simulink model "SF104A_MotCurrRegCfg"  (R2013b)
settings: Solver=FixedStepDiscrete  SolverMode=SingleTasking  StartTime=0.0  StopTime=1  FixedStep=0.002  RelTol=1e-3
values from neighbouring files (symbols this model uses):
  ARCHGLBPRM_2MILLISEC_SEC_F32 = DataDict.Constant    [SF104A_MotCurrRegCfg_DataDict.m]
  ARCHGLBPRM_2PI_ULS_F32 = DataDict.Constant    [SF104A_MotCurrRegCfg_DataDict.m]
  ARCHGLBPRM_HALFSQRT3_ULS_F32 = DataDict.Constant    [SF104A_MotCurrRegCfg_DataDict.m]
  MotCurrRegCfgCtrlrDynGainVehSpdCutOff = DataDict.Calibration    [SF104A_MotCurrRegCfg_DataDict.m]
  MotCurrRegCfgCurrLoopSecOrderTrfFctEna = DataDict.Calibration    [SF104A_MotCurrRegCfg_DataDict.m]
  MotCurrRegCfgIntglGainSampleTi = DataDict.Calibration    [SF104A_MotCurrRegCfg_DataDict.m]
  MotCurrRegCfgMotAgCompuDly = DataDict.Calibration    [SF104A_MotCurrRegCfg_DataDict.m]
  MotCurrRegCfgMotClsdLoopBwDaxY = DataDict.Calibration    [SF104A_MotCurrRegCfg_DataDict.m]
  MotCurrRegCfgMotClsdLoopBwQaxY = DataDict.Calibration    [SF104A_MotCurrRegCfg_DataDict.m]
  MotCurrRegCfgMotDampgRatDax = DataDict.Calibration    [SF104A_MotCurrRegCfg_DataDict.m]
  MotCurrRegCfgMotDampgRatQax = DataDict.Calibration    [SF104A_MotCurrRegCfg_DataDict.m]
  MotCurrRegCfgMotNatFrqDaxY = DataDict.Calibration    [SF104A_MotCurrRegCfg_DataDict.m]
  MotCurrRegCfgMotNatFrqQaxY = DataDict.Calibration    [SF104A_MotCurrRegCfg_DataDict.m]
  MotCurrRegCfgMotRVirtDax = DataDict.Calibration    [SF104A_MotCurrRegCfg_DataDict.m]
  MotCurrRegCfgMotRVirtQax = DataDict.Calibration    [SF104A_MotCurrRegCfg_DataDict.m]
  MOTDAMPGRATCON_ULS_F32 = DataDict.Constant    [SF104A_MotCurrRegCfg_DataDict.m]
  MotRefMdlFbCtrlDi = DataDict.ImprtdCal    [SF104A_MotCurrRegCfg_DataDict.m]
  POLETOPHA_ULS_F32 = DataDict.Constant    [SF104A_MotCurrRegCfg_DataDict.m]
  SysGlbPrmMotPoleCnt = DataDict.ImprtdCal    [SF104A_MotCurrRegCfg_DataDict.m]
  ZEROMOTCTRLGAIN_OHM_F32 = DataDict.Constant    [SF104A_MotCurrRegCfg_DataDict.m]
undefined symbols (not defined in the file or in its folder): MotCurrEolCalSt2
libraries: NxtrLim x11, FixdToFloat x4, LnrIntrpn x4, simulink x3, Fil x2, FloatToFixd x1
(part 3 of 3)

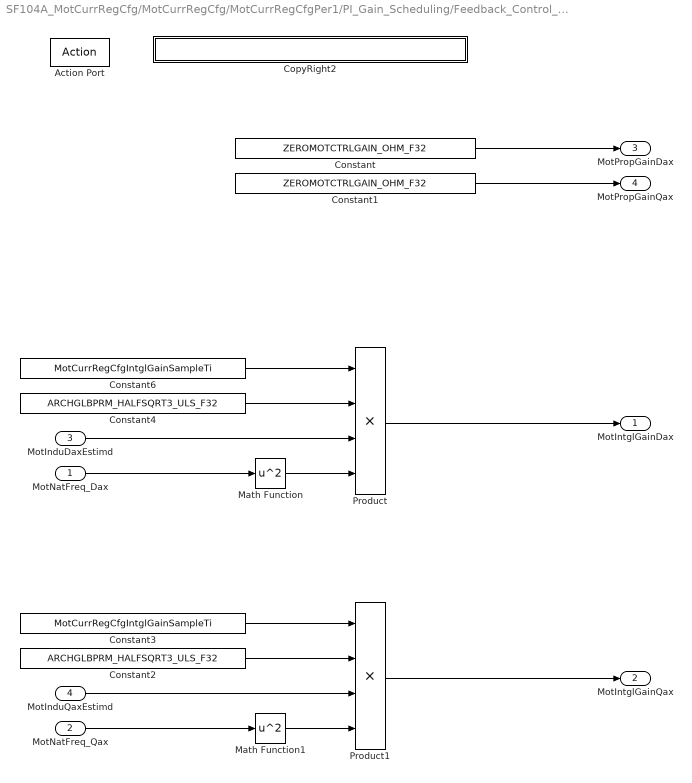
== system SF104A_MotCurrRegCfg/MotCurrRegCfg/MotCurrRegCfgPer1/PI_Gain_Scheduling/Feedback_Control_ Enabled/Calculate_Gains/2nd Order Enabled ==
  MotNatFreq_Dax : Inport  RequirementInfo="{'linktype_rmi_doors' '0000bb43 (/E-STEER Core/SubSystem Specifications/Application Functions/SF99/SF104A Current Regulator Configuration)' '#SF104A_102' 'true' 'REQ:  SF104A_102' '' } %GIDa_3ffef093_6233_4daa_8141_5ade26bfe0b7"
  MotNatFreq_Qax : Inport  RequirementInfo="{'linktype_rmi_doors' '0000bb43 (/E-STEER Core/SubSystem Specifications/Application Functions/SF99/SF104A Current Regulator Configuration)' '#SF104A_102' 'true' 'REQ:  SF104A_102' '' } %GIDa_0729f0b0_64c3_4f7f_a23b_323a26491a45"  Port=2
  MotInduDaxEstimd : Inport  RequirementInfo="{'linktype_rmi_doors' '0000bb43 (/E-STEER Core/SubSystem Specifications/Application Functions/SF99/SF104A Current Regulator Configuration)' '#SF104A_102' 'true' 'REQ:  SF104A_102' '' } %GIDa_89f11cc6_5f7a_4c49_9846_35a9922d5407"  Port=3
  MotInduQaxEstimd : Inport  RequirementInfo="{'linktype_rmi_doors' '0000bb43 (/E-STEER Core/SubSystem Specifications/Application Functions/SF99/SF104A Current Regulator Configuration)' '#SF104A_102' 'true' 'REQ:  SF104A_102' '' } %GIDa_2fe3e424_844e_4ee7_a315_46d12420253b"  Port=4
  Action Port : ActionPort  ActionType=then
  Constant : Constant  RequirementInfo="{'linktype_rmi_doors' '0000bb43 (/E-STEER Core/SubSystem Specifications/Application Functions/SF99/SF104A Current Regulator Configuration)' '#SF104A_102' 'true' 'REQ:  SF104A_102' '' } %GIDa_5901fc89_50da_4871_894f_d7a4bc965ae3"  Value=ZEROMOTCTRLGAIN_OHM_F32  OutDataTypeStr=single
  Constant1 : Constant  RequirementInfo="{'linktype_rmi_doors' '0000bb43 (/E-STEER Core/SubSystem Specifications/Application Functions/SF99/SF104A Current Regulator Configuration)' '#SF104A_102' 'true' 'REQ:  SF104A_102' '' } %GIDa_5a773f90_f553_49c4_87dd_9299d647398d"  Value=ZEROMOTCTRLGAIN_OHM_F32  OutDataTypeStr=single
  Constant2 : Constant  RequirementInfo="{'linktype_rmi_doors' '0000bb43 (/E-STEER Core/SubSystem Specifications/Application Functions/SF99/SF104A Current Regulator Configuration)' '#SF104A_102' 'true' 'REQ:  SF104A_102' '' } %GIDa_a4f8ec7f_a439_41cb_b2c0_2d5eeb2fedbe"  Value=ARCHGLBPRM_HALFSQRT3_ULS_F32
  Constant3 : Constant  RequirementInfo="{'linktype_rmi_doors' '0000bb43 (/E-STEER Core/SubSystem Specifications/Application Functions/SF99/SF104A Current Regulator Configuration)' '#SF104A_118' 'true' 'REQ:  SF104A_118' '' ; 'linktype_rmi_doors' '0000bb43 (/E-STEER Core/SubSystem Specifications/Application Functions/SF99/SF104A Current Regulator Configuration)' '#SF104A_102' 'true' 'REQ:  SF104A_102' '' } %GIDa_714edeba_1674_4f10_b7a8_b0e92a37ae0d"  Value=MotCurrRegCfgIntglGainSampleTi
  Constant4 : Constant  RequirementInfo="{'linktype_rmi_doors' '0000bb43 (/E-STEER Core/SubSystem Specifications/Application Functions/SF99/SF104A Current Regulator Configuration)' '#SF104A_102' 'true' 'REQ:  SF104A_102' '' } %GIDa_0619ee1d_6818_4fb5_9ced_1ceae65db526"  Value=ARCHGLBPRM_HALFSQRT3_ULS_F32
  Constant6 : Constant  RequirementInfo="{'linktype_rmi_doors' '0000bb43 (/E-STEER Core/SubSystem Specifications/Application Functions/SF99/SF104A Current Regulator Configuration)' '#SF104A_118' 'true' 'REQ:  SF104A_118' '' ; 'linktype_rmi_doors' '0000bb43 (/E-STEER Core/SubSystem Specifications/Application Functions/SF99/SF104A Current Regulator Configuration)' '#SF104A_102' 'true' 'REQ:  SF104A_102' '' } %GIDa_74bbab2c_1820_4b50_bb92_f8a47de750d3"  Value=MotCurrRegCfgIntglGainSampleTi
  CopyRight2 : Subsystem  Description=|  mask(Copyright Information){none=on}
      | Copyright info block.                                               
      |                                                                     
      | Place copyright information at the top of every subsystem in design.
      mask prompts: none "No parameters"
      mask help: Place copyright information at the top of every subsystem in design.
      mask Display:
      | NxtrConf = 'Nexteer Confidential';
      | 
      | sys = bdroot; %handle for the current model ("system")
      | first = get_param(sys,'Created');
      | if(isempty(first))
      |     first = datestr(now,'yyyy');
      | else
      |     first = first(end-3:end);  %year is last four digits
      | end
      | 
      | last = get_param(sys,'LastModifiedDate');
      | if isempty(last)
      |     last = datestr(now,'yyyy');
      | else
      |     last = last(end-3:end);
      | end
      | 
      | if strcmp(first,last)
      |     fprintf('%s -- Copyright %s Nexteer',NxtrConf,first)
      | else
      |     fprintf('%s -- %s%s- %s Nexteer',NxtrConf,char(169),first,last)
      | end
  Math Function : Math  RequirementInfo="{'linktype_rmi_doors' '0000bb43 (/E-STEER Core/SubSystem Specifications/Application Functions/SF99/SF104A Current Regulator Configuration)' '#SF104A_102' 'true' 'REQ:  SF104A_102' '' } %GIDa_143d8f1f_3ae5_49ad_a7bb_3d41dece4b19"  Operator=square  SaturateOnIntegerOverflow=on
  Math Function1 : Math  RequirementInfo="{'linktype_rmi_doors' '0000bb43 (/E-STEER Core/SubSystem Specifications/Application Functions/SF99/SF104A Current Regulator Configuration)' '#SF104A_102' 'true' 'REQ:  SF104A_102' '' } %GIDa_45c36ca7_c28b_4851_8d48_4fd45e280948"  Operator=square  SaturateOnIntegerOverflow=on
  Product : Product  RequirementInfo="{'linktype_rmi_doors' '0000bb43 (/E-STEER Core/SubSystem Specifications/Application Functions/SF99/SF104A Current Regulator Configuration)' '#SF104A_118' 'true' 'REQ:  SF104A_118' '' ; 'linktype_rmi_doors' '0000bb43 (/E-STEER Core/SubSystem Specifications/Application Functions/SF99/SF104A Current Regulator Configuration)' '#SF104A_102' 'true' 'REQ:  SF104A_102' '' } %GIDa_c5bd39f7_948b_46da_8578_94a785888d45"  Inputs=4
  Product1 : Product  RequirementInfo="{'linktype_rmi_doors' '0000bb43 (/E-STEER Core/SubSystem Specifications/Application Functions/SF99/SF104A Current Regulator Configuration)' '#SF104A_118' 'true' 'REQ:  SF104A_118' '' ; 'linktype_rmi_doors' '0000bb43 (/E-STEER Core/SubSystem Specifications/Application Functions/SF99/SF104A Current Regulator Configuration)' '#SF104A_102' 'true' 'REQ:  SF104A_102' '' } %GIDa_53633e1c_f6fc_4996_a26c_997da71e0e1d"  Inputs=4
  MotIntglGainDax : Outport  RequirementInfo="{'linktype_rmi_doors' '0000bb43 (/E-STEER Core/SubSystem Specifications/Application Functions/SF99/SF104A Current Regulator Configuration)' '#SF104A_102' 'true' 'REQ:  SF104A_102' '' } %GIDa_680b10bc_4fb7_47a2_8026_a2535639f1f7"
  MotIntglGainQax : Outport  RequirementInfo="{'linktype_rmi_doors' '0000bb43 (/E-STEER Core/SubSystem Specifications/Application Functions/SF99/SF104A Current Regulator Configuration)' '#SF104A_102' 'true' 'REQ:  SF104A_102' '' } %GIDa_f986541b_0aed_4a1a_957d_b7fb047d63c0"  Port=2
  MotPropGainDax : Outport  RequirementInfo="{'linktype_rmi_doors' '0000bb43 (/E-STEER Core/SubSystem Specifications/Application Functions/SF99/SF104A Current Regulator Configuration)' '#SF104A_102' 'true' 'REQ:  SF104A_102' '' } %GIDa_1ebb785c_7ee9_4c7b_9071_ad944c0df15e"  Port=3
  MotPropGainQax : Outport  RequirementInfo="{'linktype_rmi_doors' '0000bb43 (/E-STEER Core/SubSystem Specifications/Application Functions/SF99/SF104A Current Regulator Configuration)' '#SF104A_102' 'true' 'REQ:  SF104A_102' '' } %GIDa_f68b172b_2bea_4708_969a_b71eb1497900"  Port=4
  wires:
  Constant/1 -> MotPropGainDax/1
  Constant1/1 -> MotPropGainQax/1
  Product/1 -> MotIntglGainDax/1
  Math Function/1 -> Product/4
  MotNatFreq_Dax/1 -> Math Function/1
  Math Function1/1 -> Product1/4
  MotNatFreq_Qax/1 -> Math Function1/1
  MotInduQaxEstimd/1 -> Product1/3
  Product1/1 -> MotIntglGainQax/1
  MotInduDaxEstimd/1 -> Product/3
  Constant2/1 -> Product1/2
  Constant4/1 -> Product/2
  Constant6/1 -> Product/1
  Constant3/1 -> Product1/1

== system SF104A_MotCurrRegCfg/MotCurrRegCfg/MotCurrRegCfgPer1/PI_Gain_Scheduling/Feedback_Control_ Enabled/Calculate_Gains/CopyRight2 ==

== system SF104A_MotCurrRegCfg/MotCurrRegCfg/MotCurrRegCfgPer1/PI_Gain_Scheduling/Feedback_Control_ Enabled/Use_Lookup_Table/CopyRight2 ==

== system SF104A_MotCurrRegCfg/MotCurrRegCfg/MotCurrRegCfgPer1/PI_Gain_Scheduling/Feedback_Control_ Enabled/Use_Max/CopyRight2 ==

== system SF104A_MotCurrRegCfg/MotCurrRegCfg/MotCurrRegCfgPer1/PI_Gain_Scheduling/Feedback_Control_ Enabled/Calculate_Gains/2nd Order Disabled/CopyRight2 ==

== system SF104A_MotCurrRegCfg/MotCurrRegCfg/MotCurrRegCfgPer1/PI_Gain_Scheduling/Feedback_Control_ Enabled/Calculate_Gains/2nd Order Enabled/CopyRight2 ==
